simulink model "State_BS"  (R2020a)
settings: Solver=VariableStepAuto  StartTime=0.0  StopTime=10.0  RelTol=1e-3
settings Model: EnablePacing=on  Creator=wghaotian  LastModifiedBy=wghaotian

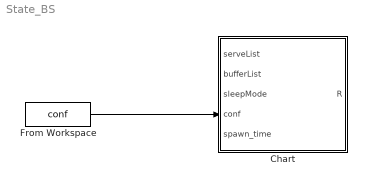
== system State_BS ==
  Chart : Stateflow chart  TreatAsAtomicUnit=on
  From Workspace : FromWorkspace  VariableName=conf
  wires:
  From Workspace/1 -> Chart/4(conf)

== stateflow chart State_BS/Chart ==
  state active
    entry:
    delay=sum(t-spawn_time(bufferList));
    R=conf.eta*energy_con+(1-conf.eta)*delay;%Cost Function, to be minimized
    serveList=bufferList;
    during:
    for usr=serveList
    % To be continued......
    % Serve the users
    end
  state SM3_deact
    entry:
    sleepMode=4;
    n=ones(3);%Action, will be implemented with eps-greedy.
    energy_con=0;%Energy consumption
    delay=0;% Delay
    t0=t;%Current time
  state Idle
    entry:
    t0=t;
    exit:
    energy_con=energy_con+(t-t0)*conf.pow_cons(1)
  state SM3_act
    exit:
    energy_con=energy_con+(t-t0)*conf.pow_cons(4);
  state SM3
  state SM2
    entry:
    sleepMode=3;
    t0=t;
  state SM1_act
    exit:
    energy_con=energy_con+(t-t0)*conf.pow_cons(2);
  state SM2_act
    exit:
    energy_con=energy_con+(t-t0)*conf.pow_cons(3);
  state SM1
    entry:
    sleepMode=2;
    t0=t;
  SM1_act -> active [order 2] : [after(conf.act_dur(2),sec)&&size(bufferList)>0]
  active -> SM3_deact : [size(serveList,1)==0]
  (default) -> SM3_deact
  SM3_act -> active [order 2] : [size(bufferList,1)>0]
  Idle -> active : [size(serveList,1)>0]
  SM2_act -> active [order 1] : [after(conf.act_dur(3),sec)&&size(bufferList)>0]
  SM3_deact -> SM3 : after(conf.deact_dur(3),sec)
  SM1_act -> Idle [order 1] : [after(conf.act_dur(2),sec)&&size(bufferList)==0]
  SM3 -> SM3 [order 2] : [after(conf.sleep_dur(4),sec)&&size(bufferList)==0]
  SM3 -> SM3_act [order 1] : [after(n(3),tick)||size(bufferList,1)>1]
  SM3_act -> SM2 [order 1] : [size(bufferList,1)==0]
  SM2 -> SM2_act [order 1] : [after(n(2),tick)||size(bufferList)>0]
  SM2 -> SM2 [order 2] : after(conf.sleep_dur(3),sec)
  SM1 -> SM1_act [order 1] : [after(n(1),tick)||size(bufferList)>0]
  SM2_act -> SM1 [order 2] : [after(conf.act_dur(3),sec)&&size(bufferList)==0]
  SM1 -> SM1 [order 2] : after(conf.sleep_dur(2),sec)
  data: n local; delay local; energy_con local; serveList input; bufferList input; sleepMode input; t0 local; conf input; spawn_time input; R output; usr local
